simulink model "deadReckoning_heading_VEX"  (R2017a)
settings: Solver=FixedStepAuto  StartTime=0.0  StopTime=10  FixedStep=Ts  RelTol=1e-3  EnableMultiTasking=on
InitFcn:
  | Ts = 0.01;
  | axleLength = 0.28;
  | wheelR = 0.052;
  | ticksPerDeg = 627.2/360;
  | load wheelMotorModel
  | load wheelMotorLUT
undefined symbols (not defined in the file): ticksPerRot
libraries: vexarmcortexlib x4, simulink_extras x1, mobileRoboticsTrainingLib x1
settings Model: ExtModeTrigDuration=25  Creator=sseshadr  LastModifiedBy=shiremat
settings OptimizationCC: PassReuseOutputArgsAs=Individual arguments  MaxStackSize=64
settings DebuggingCC: ParameterTunabilityLossMsg=error
settings HardwareCC: ProdBitPerPointer=32  ProdBitPerSizeT=32  ProdBitPerPtrDiffT=32  ProdLargestAtomicInteger=Long  ProdLargestAtomicFloat=Double  ProdWordSize=32  ProdHWDeviceType=ARM Compatible->ARM Cortex
settings SFSimCC: MATLABDynamicMemAlloc=off
settings RTWCC: SystemTargetFile=ert.tlc  HardwareBoard=ARM Cortex-based VEX Microcontroller  TLCOptions="-aInlineSetEventsForThisBaseRateFcn=TLC_FALSE -aSuppressMultiTaskScheduler=TLC_FALSE  -aRateBasedStepFcn=0"  TemplateMakefile=ert_default_tmf  Description=Embedded Coder  GenerateReport=on  Toolchain=GNU Tools for VEX ARM Cortex  IncludeHyperlinkInReport=on  LaunchReport=on  GenerateTraceInfo=on  GenerateTraceReport=on  GenerateTraceReportSl=on  GenerateTraceReportSf=on  GenerateTraceReportEml=on
settings CodeAppCC: ForceParamTrailComments=on  IgnoreCustomStorageClasses=off  OperatorAnnotations=on  SimulinkDataObjDesc=on  SFDataObjDesc=on  MATLABFcnDesc=on  InsertBlockDesc=on  MATLABSourceComments=on

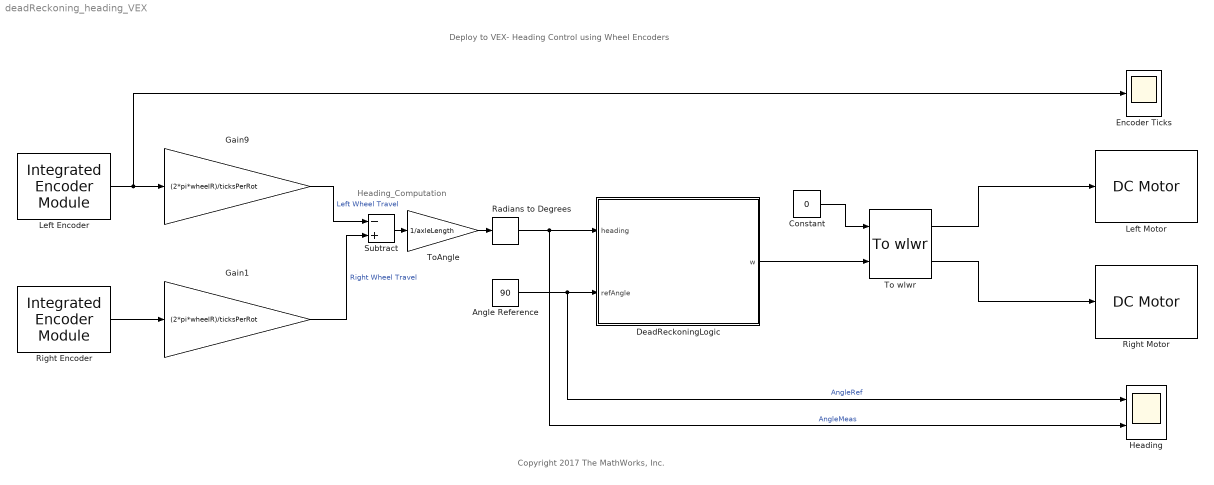
== system deadReckoning_heading_VEX ==
  note: Deploy to VEX- Heading Control using Wheel Encoders
  note: Heading_Computation
  note: Copyright 2017 The MathWorks, Inc.
  Angle Reference : Constant  Value=90
  Constant : Constant  Value=0
  DeadReckoningLogic : Stateflow chart  TreatAsAtomicUnit=on
  Encoder Ticks : Scope
  Gain1 : Gain  Gain=(2*pi*wheelR)/ticksPerRot
  Gain9 : Gain  Gain=(2*pi*wheelR)/ticksPerRot
  Heading : Scope  NumInputPorts=2
  Left Encoder : vexarmcortexlib/Sensors/Integrated Encoder Module  motorType=VEX 393 (High torque)  seqNumI2C=1  resetOption=No reset  rotVelocity=off  inputPortSim=off  SampleTime=Ts
      settings: SourceProductName=Simulink Coder Support Package for ARM Cortex-based VEX Microcontroller  SourceProductBaseCode=EC_VEX_MICRO
  Left Motor : vexarmcortexlib/Actuators/DC Motor  motor=10  scaleFactor=1/13.5  SimulationOut=off
      settings: SourceProductName=Simulink Coder Support Package for ARM Cortex-based VEX Microcontroller  SourceProductBaseCode=EC_VEX_MICRO
  Radians to Degrees : simulink_extras/Transformations/Radians to Degrees
  Right Encoder : vexarmcortexlib/Sensors/Integrated Encoder Module  motorType=VEX 393 (High torque)  seqNumI2C=0  resetOption=No reset  rotVelocity=off  inputPortSim=off  SampleTime=Ts
      settings: SourceProductName=Simulink Coder Support Package for ARM Cortex-based VEX Microcontroller  SourceProductBaseCode=EC_VEX_MICRO
  Right Motor : vexarmcortexlib/Actuators/DC Motor  motor=1  scaleFactor=1/13.5  SimulationOut=off
      settings: SourceProductName=Simulink Coder Support Package for ARM Cortex-based VEX Microcontroller  SourceProductBaseCode=EC_VEX_MICRO
  Subtract : Sum  Inputs=-+
  To wlwr : mobileRoboticsTrainingLib/To wlwr  axleLength=0.1  wheelR=0.05
  ToAngle : Gain  Gain=1/axleLength
  wires:
  Radians to Degrees/1 -> Heading/2, DeadReckoningLogic/1(heading)  "AngleMeas"
  Gain9/1 -> Subtract/1  "Left Wheel Travel"
  Subtract/1 -> ToAngle/1
  Gain1/1 -> Subtract/2  "Right Wheel Travel"
  Left Encoder/1 -> Encoder Ticks/1, Gain9/1
  Right Encoder/1 -> Gain1/1
  To wlwr/1 -> Left Motor/1
  To wlwr/2 -> Right Motor/1
  Angle Reference/1 -> Heading/1, DeadReckoningLogic/2(refAngle)  "AngleRef"
  ToAngle/1 -> Radians to Degrees/1
  DeadReckoningLogic/1(w) -> To wlwr/2
  Constant/1 -> To wlwr/1

== stateflow chart deadReckoning_heading_VEX/DeadReckoningLogic ==
  state Rotate
    entry:
    w = 1;
  state Stop
    entry:
    w = 0;
  (default) -> Rotate : %Start Dead Reckoning
  Rotate -> Stop : [heading >= refAngle]
  data: heading input; w output; refAngle input
